simulink model "Subsytem"  (R2020b)
settings: Solver=FixedStepAuto  StartTime=0.0  StopTime=10.0  FixedStep=0.2  RelTol=1e-3
settings Model: Creator=varunraj  LastModifiedBy=varunraj
settings DataIOCC: SaveOutput=off  SaveTime=off

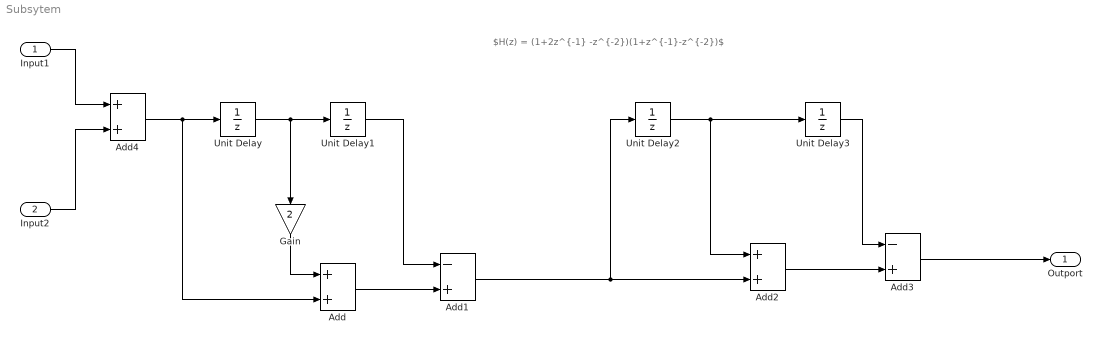
== system Subsytem ==
  note: $H(z) = (1+2z^{-1} -z^{-2})(1+z^{-1}-z^{-2})$
  Input1 : Inport  OutDataTypeStr=double  PortDimensions=1  SampleTime=[0.20000000000000001,0]
  Input2 : Inport  Port=2  OutDataTypeStr=double  PortDimensions=1  SampleTime=[0.20000000000000001,0]
  Add : Sum
  Add1 : Sum  Inputs=-+
  Add2 : Sum
  Add3 : Sum  Inputs=-+
  Add4 : Sum
  Gain : Gain  Gain=2
  Unit Delay{,1..3} (4 alike) : UnitDelay  SampleTime=-1  HasFrameUpgradeWarning=on
  Outport : Outport  OutDataTypeStr=double  PortDimensions=1  SampleTime=[0.20000000000000001,0]
  wires:
  Gain/1 -> Add/1
  Add4/1 -> Unit Delay/1, Add/2
  Add2/1 -> Add3/2
  Input2/1 -> Add4/2
  Add3/1 -> Outport/1
  Add1/1 -> Add2/2, Unit Delay2/1
  Unit Delay/1 -> Unit Delay1/1, Gain/1
  Unit Delay1/1 -> Add1/1
  Unit Delay2/1 -> Add2/1, Unit Delay3/1
  Input1/1 -> Add4/1
  Unit Delay3/1 -> Add3/1
  Add/1 -> Add1/2
